simulink model "ssc_car_fuel_cell_1motor"  (R2026a)
settings: Solver=daessc  StopTime=195  FixedStep=1e-3  AbsTol=1e-3
InitFcn:
  | %Vehicle = sm_car_vehcfg_checkConfig(Vehicle);
undefined symbols (not defined in the file): Control, Driver, Init, Maneuver1, Vehicle
libraries: fl_lib x93, nesl_utility x38, GasN_lib x21, sdl_lib x10, simulink_extras x6, SimscapeFluids_lib x6, simulink x5, customMath_lib x5, slpidlib x4, ee_lib x3, autolibshared x2, sl_discontinuities x2
(part 1 of 4)
Description:
  | Vehicle with Fuel Cell Powertrain
  | 
  | Copyright 2020-2025 The MathWorks, Inc.
settings Model: PauseTimes=10  Creator=jrodgers  LastModifiedBy=smiller
settings SolverCC: MaxConsecutiveMinStep=5  SolverJacobianMethodControl=SparsePerturbation  DaesscMode=Fast
settings DataIOCC: SaveFormat=StructureWithTime  SignalLoggingName=logsout_ssc_FuelCell1Motor  ReturnWorkspaceOutputsName=dataOut
settings DebuggingCC: IgnoredZcDiagnostic=none
settings SimscapeCC: SimscapeNominalValues="[{\"value\":\"1\",\"unit\":\"A\"},{\"value\":\"1\",\"unit\":\"bar\"},{\"value\":\"1\",\"unit\":\"cm^2\"},{\"value\":\"1\",\"unit\":\"cm^3/s\"},{\"value\":\"5e6\",\"unit\":\"J/kg\"},{\"value\":\"1\",\"unit\":\"kW\"},{\"value\":\"1\",\"unit\":\"l\"},{\"value\":\"1\",\"unit\":\"N\"},{\"value\":\"1\",\"unit\":\"N*m\"},{\"value\":\"400\",\"unit\":\"V\"},{\"value\":\"355\",\"unit\":\"K\"}]"  SimscapeLogSimulationStatistics=on  SimscapeLogName=simlog_ssc_FuelCell1Motor  SimscapeLogLimitData=off  SimscapeLogDataHistory=5000.0  SimscapeOperatingPoint=ssc_FuelCell1Motor_op10sec

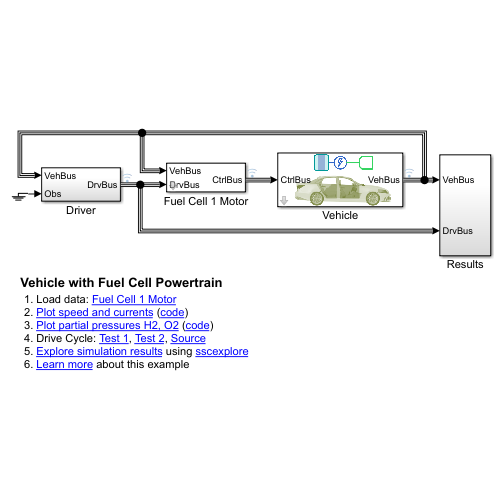
[thumbnail: Simulink's stored preview of the top-level diagram]
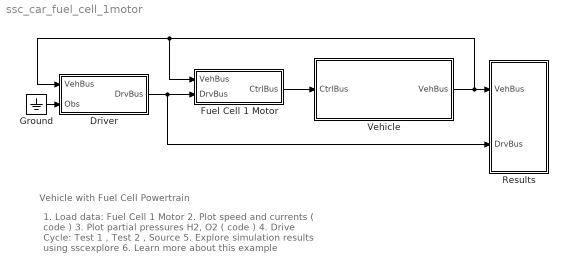
== system ssc_car_fuel_cell_1motor ==
  note: Vehicle with Fuel Cell Powertrain
  note: 1. Load data: Fuel Cell 1 Motor
      | 2. Plot speed and currents ( code )
      | 3. Plot partial pressures H2, O2 ( code )
      | 4. Drive Cycle: Test 1 , Test 2 , Source
      | 5. Explore simulation results using sscexplore
      | 6. Learn more about this example
  Driver : Subsystem  VariantControl=Drive_Cycle
  Fuel Cell 1 Motor : Subsystem  VariantControl=FuelCell1Motor  mask(Control of Fuel Cell Powertrain){Control=Control.FuelCell1Motor}
      mask prompts: Control "Control (structure)"
      mask help: Models control algorithm for fuel cell and regenerative braking of single motor powertrain.
  Ground : Ground
  Results : Subsystem
  Vehicle : Subsystem  mask{Vehicle=Vehicle}
      mask prompts: Vehicle "Vehicle (Structure)"
      mask Display: image('ssc_vehicle_fuel_cell_1motor_vehicle_IMAGE.png');
  wires:
  Vehicle/1(VehBus) -> Fuel Cell 1 Motor/1(VehBus), Driver/1(VehBus), Results/1(VehBus)
  Fuel Cell 1 Motor/1(CtrlBus) -> Vehicle/1(CtrlBus)
  Ground/1 -> Driver/2(Obs)
  Driver/1(DrvBus) -> Fuel Cell 1 Motor/2(DrvBus), Results/2(DrvBus)

== system ssc_car_fuel_cell_1motor/Driver ==
  In Bus Element : Inport  PortName=VehBus  Element=Chassis.Body.CG.vx
  Obs : Inport  Port=2
  Bus Creator2 : BusCreator  Inputs=4
  Constant1 : Constant  Value=0
  Drive Cycle : Subsystem  Variant=on  VariantControlMode=label  VariantControl=Choice  LabelModeActiveChoice=Data
      settings: AttributesFormatString=%<LabelModeActiveChoice>
      mask Display: disp(' ');
  Reference : Subsystem
  Terminator1 : Terminator
  Vehicle Speed Controller : Subsystem  Variant=on  VariantControlMode=label  VariantControl=Choice  LabelModeActiveChoice=Ideal  mask(Driver Model){popup_drivertype=Ideal}
      mask prompts: popup_drivertype "Driver Type"
      mask help: Select from two options. "Ideal" is a simple PI controller. "Configurable" uses the Longitudinal Driver block from Powertrain Blockset which can be configured to include more advanced driver behavior.
      mask init:
      | set_param(gcb,'LabelModeActiveChoice',get_param(gcb,'popup_drivertype'));
      settings: AttributesFormatString=%<LabelModeActiveChoice>
      mask TypeOptions popup_drivertype: Ideal | Configurable
  DrvBus : Outport  VectorParamsAs1DForOutWhenUnconnected=off
  wires:
  Reference/1(Ref) -> Bus Creator2/1  "Reference"
  Constant1/1 -> Bus Creator2/4  "aSteerWheel"
  Bus Creator2/1 -> DrvBus/1
  Obs/1 -> Terminator1/1
  Drive Cycle/1(Reference Speed) -> Reference/1(vTarget), Vehicle Speed Controller/1(Ref Spd)  "vTarget"
  In Bus Element/1 -> Vehicle Speed Controller/2(Veh Spd)
  Vehicle Speed Controller/1(rBrakePedal) -> Bus Creator2/2
  Vehicle Speed Controller/2(rAccelPedal) -> Bus Creator2/3

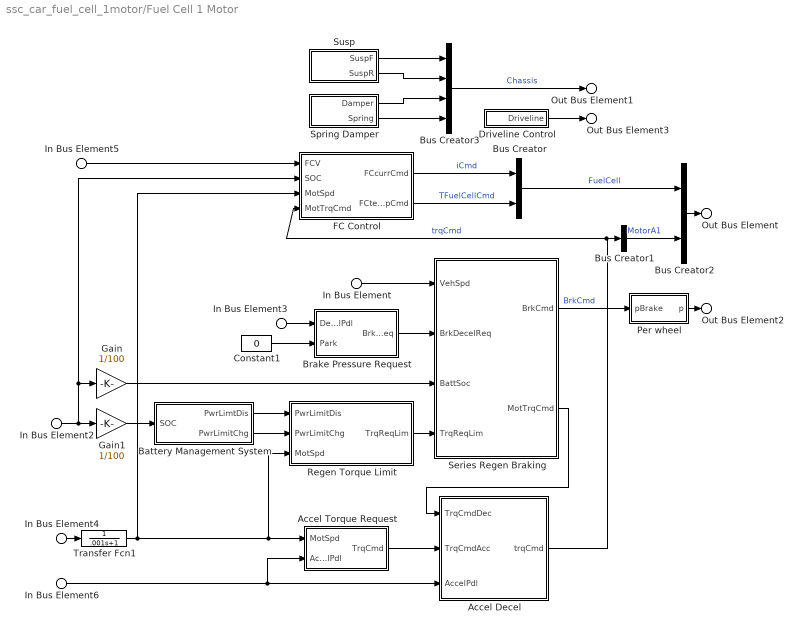
== system ssc_car_fuel_cell_1motor/Fuel Cell 1 Motor ==
  In Bus Element : Inport  PortName=VehBus  Element=Chassis.Body.CG.vx
  In Bus Element2 : Inport  PortName=VehBus  Element=Power.Battery.SOC
  In Bus Element5 : Inport  PortName=VehBus  Element=Power.FuelCell.v
  In Bus Element4 : Inport  PortName=VehBus  Element=Power.MotorA1.w
  In Bus Element3 : Inport  Port=2  PortName=DrvBus  Element=rBrakePedal
  In Bus Element6 : Inport  Port=2  PortName=DrvBus  Element=rAccelPedal
  Accel Decel : Subsystem
  Accel Torque Request : Subsystem
  Battery Management System : Subsystem
  Brake Pressure Request : Subsystem
  Bus Creator : BusCreator  Inputs=2
  Bus Creator1 : BusCreator  Inputs=1
  Bus Creator2 : BusCreator  Inputs=2
  Bus Creator3 : BusCreator  Inputs=4
  Constant1 : Constant  Value=0
  Driveline Control : Subsystem
  FC Control : Subsystem
  Gain : Gain  Gain=1/100
  Gain1 : Gain  Gain=1/100
  Per wheel : Subsystem
  Regen Torque Limit : Subsystem
  Series Regen Braking : Subsystem  InitFcn=%[~]=autosharedicon('autolibutils',gcb,0);  VariantControl=Variant
  Spring Damper : Subsystem
  Susp : Subsystem
  Transfer Fcn1 : TransferFcn  Denominator=[.001 1]
  Out Bus Element : Outport  PortName=CtrlBus  Element=Power
  Out Bus Element2 : Outport  PortName=CtrlBus  Element=Brakes
  Out Bus Element1 : Outport  PortName=CtrlBus  Element=Chassis
  Out Bus Element3 : Outport  PortName=CtrlBus  Element=Driveline
  wires:
  Battery Management System/2(PwrLimitChg) -> Regen Torque Limit/2("PwrLimitChg ")
  Battery Management System/1(PwrLimtDis) -> Regen Torque Limit/1(PwrLimitDis)
  Brake Pressure Request/1(BrkDecelReq) -> Series Regen Braking/2(BrkDecelReq)
  Constant1/1 -> Brake Pressure Request/2(Park)
  In Bus Element/1 -> Series Regen Braking/1(VehSpd)
  Regen Torque Limit/1("TrqReqLim ") -> Series Regen Braking/4(TrqReqLim)
  Accel Torque Request/1(TrqCmd) -> Accel Decel/2(TrqCmdAcc)
  Per wheel/1(p) -> Out Bus Element2/1
  Series Regen Braking/1(" BrkCmd") -> Per wheel/1(pBrake)  "BrkCmd"
  Series Regen Braking/2(" MotTrqCmd") -> Accel Decel/1(TrqCmdDec)
  Driveline Control/1(Driveline) -> Out Bus Element3/1
  Susp/2(SuspR) -> Bus Creator3/2
  Spring Damper/2(Spring) -> Bus Creator3/4
  Bus Creator3/1 -> Out Bus Element1/1  "Chassis"
  Susp/1(SuspF) -> Bus Creator3/1
  Spring Damper/1(Damper) -> Bus Creator3/3
  Transfer Fcn1/1 -> FC Control/3(MotSpd), Accel Torque Request/1(MotSpd), Regen Torque Limit/3(MotSpd)
  Bus Creator2/1 -> Out Bus Element/1
  Bus Creator1/1 -> Bus Creator2/2  "MotorA1"
  Bus Creator/1 -> Bus Creator2/1  "FuelCell"
  FC Control/1(FCcurrCmd) -> Bus Creator/1  "iCmd"
  In Bus Element5/1 -> FC Control/1(FCV)
  FC Control/2(FCtempCmd) -> Bus Creator/2  "TFuelCellCmd"
  In Bus Element2/1 -> Gain1/1, Gain/1, FC Control/2(SOC)
  In Bus Element3/1 -> Brake Pressure Request/1(DecelPdl)
  Gain/1 -> Series Regen Braking/3(BattSoc)
  In Bus Element4/1 -> Transfer Fcn1/1
  Gain1/1 -> Battery Management System/1(SOC)
  In Bus Element6/1 -> Accel Decel/3(AccelPdl), Accel Torque Request/2(AccelPdl)
  Accel Decel/1(trqCmd) -> Bus Creator1/1, FC Control/4(MotTrqCmd)  "trqCmd"

== system ssc_car_fuel_cell_1motor/Results ==
  In Bus Element3 : Inport  PortName=VehBus
  In Bus Element2 : Inport  PortName=VehBus  Element=Power.FuelCell.i
  In Bus Element1 : Inport  PortName=VehBus  Element=Power.Battery.Power
  DrvBus : Inport  Port=2
  Bus Selector : BusSelector  OutputSignals=Reference.vTarget
  Bus Selector1 : BusSelector  OutputSignals=Chassis.Body.CG.vx
  Fuel Economy : Subsystem
  Scope : Scope  NumInputPorts=2
      settings: ActiveDisplayYMinimum=-3.42768  ActiveDisplayYMaximum=28.54488
  Scope1 : Scope  NumInputPorts=2
      settings: ActiveDisplayYMinimum=-12.71615  ActiveDisplayYMaximum=114.44535  DataLoggingVariableName=ScopeData2
  wires:
  DrvBus/1 -> Bus Selector/1
  Bus Selector/1 -> Scope/1  "<vTarget>"
  In Bus Element3/1 -> Bus Selector1/1
  Bus Selector1/1 -> Fuel Economy/1(In1), Scope/2  "<vx>"
  In Bus Element2/1 -> Fuel Economy/2(In2)
  In Bus Element1/1 -> Fuel Economy/3(In3)
  Fuel Economy/1(MPGe) -> Scope1/1  "MPGe"
  Fuel Economy/2(l/100km) -> Scope1/2  "Liters/100km"

== system ssc_car_fuel_cell_1motor/Vehicle ==
  In Bus Element : Inport  PortName=CtrlBus  Element=Power
  In Bus Element2 : Inport  PortName=CtrlBus  Element=Brakes
  Chassis : Subsystem  VariantControl=Full
      mask Display: image('ssc_vehicle_fuel_cell_1motor_chassis_IMAGE.png');
  Powertrain : Subsystem  mask{Powertrain=Vehicle.Powertrain}
      mask prompts: Powertrain "Powertrain (structure)"
      mask Display: image('ssc_vehicle_fuel_cell_1motor_powertrain_IMAGE.png');
  Solver Configuration : nesl_utility/Solver Configuration  PhysicalDomain=network_engine_domain  SubClassName=solver  LeftPortType=input  RightPortType=generic  Tones=[]  Harmonics=[]  SimulateNoise=off  Profile=off  UseLocalSampling=off  EnableSwitchedLinearOptims=on  FrequencyDomain=off  UseCCode=off  RelTol=0.001  AbsTol=1e-06  MinStep=1e-09  ToWorkspace=off  RevertToSquareIcSolve=off  NumHomotopyIterations=100  PhasorMode=off  PhasorModeNumHarmonics=1  ConsistencySolver=NEWTON_FTOL  CanonicalOrdering=UNORDERED  OptimizeIntermediates=UNOPTIMIZED  IndexReductionMethod=DerivativeReplacement  DoDC=off  ResidualTolerance=1e-09  ConsistencyTolSource=GLOBAL  ConsistencyAbsTol=0.001  ConsistencyRelTol=0.001  ConsistencyTolFactor=0.001  UseLocalSolver=off  LocalSolverChoice=NE_BACKWARD_EULER_ADVANCER  ResolveIndetEquations=on  FunctionEvalNumThread=1  LocalSolverSampleTime=0.001  DoFixedCost=off  MaxNonlinIter=3  MaxModeIter=2  ComputeImpulses=off  ImpulseIterations=2  LinearAlgebra=auto  LinearAlgebraNumThread=0  EquationFormulation=NE_TIME_EF  DelaysMemoryBudget=1024  AutomaticFiltering=on  FilteringTimeConstant=0.001  PartitionStorageMethod=AS_NEEDED  PartitionMemoryBudget=1024  PartitionMethod=FAST  MultibodyUseLocalSolver=off  MultibodyLocalSolverChoice=ODE1  MultibodyLocalSolverSampleTime=0.001
  Out Bus Element : Outport  PortName=VehBus  Element=Power
  Out Bus Element1 : Outport  PortName=VehBus  Element=Chassis
  wires:
  Powertrain/1(OutP) -> Out Bus Element/1
  In Bus Element2/1 -> Chassis/1(Brakes)
  In Bus Element/1 -> Powertrain/2(CtrlP)
  Chassis/1(VehBus) -> Powertrain/1(VehB), Out Bus Element1/1
  connections:
  Chassis/RConn1 -- Powertrain/RConn1
  Powertrain/LConn1 -- Chassis/LConn1 -- Solver Configuration/RConn1

== system ssc_car_fuel_cell_1motor/Driver/Drive Cycle ==
  Drive Cycle Data : Subsystem  VariantControl=Data  mask{popup_cycle=Cycle 1, Drive_Cycle_Time=Maneuver1.DriveCycle.cycle_t.Value, Drive_Cycle_Speed=Maneuver1.DriveCycle.cycle_spd.Value}
      mask prompts: popup_cycle "Drive Cycle"; Drive_Cycle_Time "Drive Cycle Time (s)"; Drive_Cycle_Speed "Drive Cycle Speed (km/h)"
      mask init:
      | if(verLessThan('matlab','9.7'))
      |     set_param([gcb '/1-D Lookup Table'],'InterpMethod','Cubic spline')
      | else
      |     set_param([gcb '/1-D Lookup Table'],'InterpMethod','Akima spline')
      | end
      mask TypeOptions popup_cycle: Cycle 1 | Cycle 2 | Custom
      mask Callback popup_cycle:
      | maskObj = Simulink.Mask.get(gcb);
      | dct_h = maskObj.getParameter('Drive_Cycle_Time');
      | dcs_h = maskObj.getParameter('Drive_Cycle_Speed');
      | 
      | if strcmp(get_param(gcb,'popup_cycle'),'Cycle 1')
      |     dct_h.Value = 'Maneuver1.DriveCycle.cycle_t.Value';
      |     dcs_h.Value = 'Maneuver1.DriveCycle.cycle_spd.Value';
      |     dct_h.Enabled = 'off';
      |     dcs_h.Enabled = 'off';
      | elseif strcmp(get_param(gcb,'popup_cycle'),'Cycle 2')
      |     dct_h.Value = 'Maneuver2.DriveCycle.cycle_t.Value';
      |     dcs_h.Value = 'Maneuver2.DriveCycle.cycle_spd.Value';
      |     dct_h.Enabled = 'off';
      |     dcs_h.Enabled = 'off';
      | elseif strcmp(get_param(gcb,'popup_cycle'),'Custom')
      |     dct_h.Enabled = 'on';
      |     dcs_h.Enabled = 'on';
      | end
      | 
      | clear maskObj dct_h dcs_h
  Drive Cycle Source : autolibshared/Drive Cycle Source  VariantControl=Source  cycleVar=FTP75  fileVar=cycleFTP75.mat  tfinal="2474  seconds"  cycleRepeat=off  outAccPort=off  outGearPort=off  gearList=No gear data  t_wot1=5  xdot_woto=0  xdot_wot1=30  t_wot2=20  xdot_wot2=0  t_wotend=30  srcUnit=m/s  outUnit=m/s  srcAccUnit=m/s/s  outAccUnit=m/s^2  dt=0  aMode=1  faultOption=off  velBnd=2  velBndUnit=mph  inUnit=m/s  timeBnd=1  failOption=off  stopSim=off  maxFaultCnt=10  maxFaultTime=2  maxTotFaultTime=15  traceOption=off  dtTrace=1  traceWindow=10  lastDCname=FTP75  lastOutUnit=mph  lastDT=0  lastTB=1  lastSB=2  forceCalcBound=off
  Reference Speed : Outport

== system ssc_car_fuel_cell_1motor/Driver/Reference ==
  vTarget : Inport
  Bus Creator : BusCreator  Inputs=5
  Constant2 : Constant  Value=0
  Constant4 : Constant  Value=0
  Gain : Gain
  Integrator : Integrator
  Ref : Outport  VectorParamsAs1DForOutWhenUnconnected=off
  wires:
  Bus Creator/1 -> Ref/1
  Constant2/1 -> Bus Creator/3  "y"
  Gain/1 -> Bus Creator/1  "dist"
  Integrator/1 -> Gain/1, Bus Creator/2  "x"
  Constant4/1 -> Bus Creator/4  "aYaw"
  vTarget/1 -> Integrator/1, Bus Creator/5

== system ssc_car_fuel_cell_1motor/Driver/Vehicle Speed Controller ==
  Ref Spd : Inport
  Veh Spd : Inport  Port=2
  Configurable : Subsystem  VariantControl=Configurable
  Ideal : Subsystem  VariantControl=Ideal  mask(PI Controller){Driver=Driver}
      mask prompts: Driver "Driver (structure)"
      mask help: Simple PI controller to follow reference signal.
  rBrakePedal : Outport
  rAccelPedal : Outport  Port=2

== system ssc_car_fuel_cell_1motor/Fuel Cell 1 Motor/Accel Decel ==
  TrqCmdDec : Inport
  TrqCmdAcc : Inport  Port=2
  AccelPdl : Inport  Port=3
  Accel Decel Switch : Switch  Criteria=u2 > Threshold  SaturateOnIntegerOverflow=off  InputSameDT=off
  Compare To Constant : simulink/Logic and Bit Operations/Compare To Constant  relop=>  const=1e-3  OutDataTypeStr=boolean  ZeroCross=off
  trqCmd : Outport  VectorParamsAs1DForOutWhenUnconnected=off
  wires:
  Compare To Constant/1 -> Accel Decel Switch/2
  AccelPdl/1 -> Compare To Constant/1
  TrqCmdAcc/1 -> Accel Decel Switch/1
  Accel Decel Switch/1 -> trqCmd/1
  TrqCmdDec/1 -> Accel Decel Switch/3

== system ssc_car_fuel_cell_1motor/Fuel Cell 1 Motor/Accel Torque Request ==
  note: Convert Accelerator Pedal Position to Torque Command
      | using Motor Torque Speed Curve
  MotSpd : Inport
  AccelPdl : Inport  Port=2
  MaxMotTrqVsSpd : Lookup_n-D  NumberOfTableDimensions=1  BreakpointsForDimension1=Control.MotorA1.TorqueSpd.w.Value %Mot.w_eff_bp_EV_rear  Table=Control.MotorA1.TorqueSpd.trq.Value % Mot.T_t_EV_rear  ExtrapMethod=Clip  UseLastTableValue=on  InternalRulePriority=Speed  OutDataTypeStr=Inherit: Inherit from 'Table data'  RndMeth=Simplest
  Product1 : Product
  rads_to_rpm : Gain  Gain=30/pi
  TrqCmd : Outport  VectorParamsAs1DForOutWhenUnconnected=off
  wires:
  Product1/1 -> TrqCmd/1
  MaxMotTrqVsSpd/1 -> Product1/2
  AccelPdl/1 -> Product1/1
  MotSpd/1 -> rads_to_rpm/1
  rads_to_rpm/1 -> MaxMotTrqVsSpd/1

== system ssc_car_fuel_cell_1motor/Fuel Cell 1 Motor/Battery Management System ==
  note: Behaviorial BMS System. Limits battery charge / discharge power based on SOC.
      |
      | Charge/Discharge Limits and curves can be adjusted if using a larger battery pack
      | or motor power is changed.
  SOC : Inport
  ChrgLmt : Lookup_n-D  NumberOfTableDimensions=1  BreakpointsForDimension1=Control.Battery.SOC_bpt  Table=Control.Battery.ChrgLmt_bpt  ExtrapMethod=Clip  UseLastTableValue=on  InternalRulePriority=Speed  RndMeth=Simplest
  DischrgLmt : Lookup_n-D  NumberOfTableDimensions=1  BreakpointsForDimension1=Control.Battery.SOC_bpt  Table=Control.Battery.DischrgLmt_bpt  ExtrapMethod=Clip  UseLastTableValue=on  InternalRulePriority=Speed  RndMeth=Simplest
  MaxChrg : Constant  Value=Control.Battery.BattChrgMax
  MaxDischrg : Constant  Value=Control.Battery.BattDischrgMax
  Product : Product
  Product1 : Product
  PwrLimtDis : Outport  VectorParamsAs1DForOutWhenUnconnected=off
  PwrLimitChg : Outport  Port=2  VectorParamsAs1DForOutWhenUnconnected=off
  wires:
  SOC/1 -> DischrgLmt/1, ChrgLmt/1
  MaxChrg/1 -> Product1/2
  MaxDischrg/1 -> Product/2
  Product/1 -> PwrLimtDis/1
  Product1/1 -> PwrLimitChg/1
  ChrgLmt/1 -> Product1/1
  DischrgLmt/1 -> Product/1

== system ssc_car_fuel_cell_1motor/Fuel Cell 1 Motor/Brake Pressure Request ==
  note: Converts Brake Pedal Position to Deceleration Request
  DecelPdl : Inport
  Park : Inport  Port=2
  Constant1 : Constant
  Switch : Switch  Criteria=u2 > Threshold  ZeroCross=off  SaturateOnIntegerOverflow=off  InputSameDT=off
  BrkDecelReq : Outport  VectorParamsAs1DForOutWhenUnconnected=off
  wires:
  DecelPdl/1 -> Switch/3
  Constant1/1 -> Switch/1
  Switch/1 -> BrkDecelReq/1
  Park/1 -> Switch/2

== system ssc_car_fuel_cell_1motor/Fuel Cell 1 Motor/Driveline Control ==
  Bus Creator : BusCreator  Inputs=1
  Constant : Constant  Value=0
  Driveline : Outport  VectorParamsAs1DForOutWhenUnconnected=off
  wires:
  Constant/1 -> Bus Creator/1  "placeholder"
  Bus Creator/1 -> Driveline/1  "Driveline"

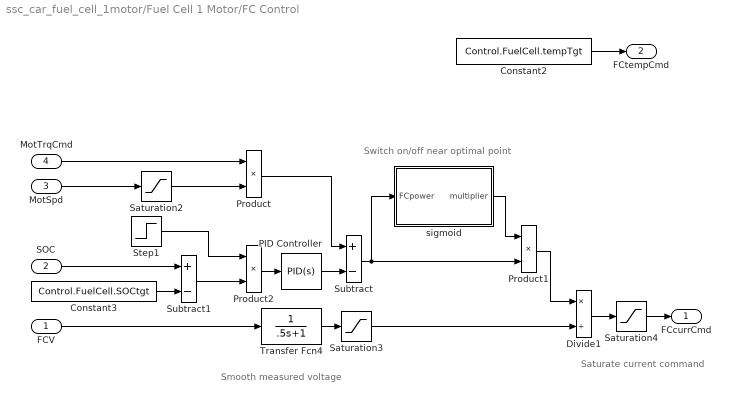
== system ssc_car_fuel_cell_1motor/Fuel Cell 1 Motor/FC Control ==
  note: Saturate current command
  note: Smooth measured voltage
  note: Switch on/off near optimal point
  FCV : Inport
  SOC : Inport  Port=2
  MotSpd : Inport  Port=3
  MotTrqCmd : Inport  Port=4
  Constant2 : Constant  Value=Control.FuelCell.tempTgt
  Constant3 : Constant  Value=Control.FuelCell.SOCtgt
  Divide1 : Product  Inputs=*/
  PID Controller : slpidlib/PID Controller  Controller=PID  Form=Parallel  TimeDomain=Continuous-time  UseExternalTs=off  SampleTime=-1  IntegratorMethod=Forward Euler  FilterMethod=Forward Euler  ControllerParametersSource=internal  P=10000/100  I=0  UseKiTs=off  D=0  UseExternalDerivativeSource=off  N=100  UseFilter=on  TunerSelectOption=Transfer Function Based (PID Tuner App)  ZeroCross=off  InitialConditionSource=internal  InitialConditionForIntegrator=0  InitialConditionForFilter=0  DifferentiatorICPrevScaledInput=0  ExternalReset=none  TrackingMode=off  Kt=1  LimitOutput=off  SatLimitsSource=internal  UpperSaturationLimit=inf  LowerSaturationLimit=-inf  LinearizeAsGain=on  AntiWindupMode=none  Kb=1  LimitIntegrator=off  UpperIntegratorSaturationLimit=inf  LowerIntegratorSaturationLimit=-inf  POutMin=[]  POutMax=[]  IOutMin=[]  IOutMax=[]  DOutMin=[]  DOutMax=[]  NOutMin=[]  NOutMax=[]  SumOutMin=[]  SumOutMax=[]  SaturationOutMin=[]  SaturationOutMax=[]  PParamMin=[]  PParamMax=[]  IParamMin=[]  IParamMax=[]  DParamMin=[]  DParamMax=[]  NParamMin=[]  NParamMax=[]  KbParamMin=[]  KbParamMax=[]  KtParamMin=[]  KtParamMax=[]  KbOutMin=[]  KbOutMax=[]  KtOutMin=[]  KtOutMax=[]  IntegratorOutMin=[]  IntegratorOutMax=[]  FilterOutMin=[]  FilterOutMax=[]  SumI1OutMin=[]  SumI1OutMax=[]  SumI2OutMin=[]  SumI2OutMax=[]  SumI3OutMin=[]  SumI3OutMax=[]  SumI4OutMin=[]  SumI4OutMax=[]  SumDOutMin=[]  SumDOutMax=[]  DifferentiatorOutMin=[]  DifferentiatorOutMax=[]  FilterDiffOutCoefMin=[]  FilterDiffOutCoefMax=[]  ReciprocalOutMin=[]  ReciprocalOutMax=[]  SumDenOutMin=[]  SumDenOutMax=[]  SumNumOutMin=[]  SumNumOutMax=[]  DivideOutMin=[]  DivideOutMax=[]  UdiffTsProdOutMin=[]  UdiffTsProdOutMax=[]  NTsProdOutMin=[]  NTsProdOutMax=[]  UintegralTsProdOutMin=[]  UintegralTsProdOutMax=[]  UngainTsProdOutMin=[]  UngainTsProdOutMax=[]  ClampingZeroOutDataTypeStr=Inherit: Inherit via back propagation  ClampingZeroOutMin=[]  ClampingZeroOutMax=[]  FilterDenConstantOutDataTypeStr=Inherit: Inherit via back propagation  FilterDenConstantOutMin=[]  FilterDenConstantOutMax=[]  PCopyOutDataTypeStr=Inherit: Inherit via back propagation  PCopyOutMin=[]  PCopyOutMax=[]  NCopyOutDataTypeStr=Inherit: Inherit via back propagation  NCopyOutMin=[]  NCopyOutMax=[]  IntegratorContinuousStateAttributes=''  IntegratorStateMustResolveToSignalObject=off  IntegratorRTWStateStorageClass=Auto  FilterContinuousStateAttributes=''  FilterStateMustResolveToSignalObject=off  FilterRTWStateStorageClass=Auto  ParallelPVariant=InternalParameters  IdealPVariant=Disabled  IVariant=InternalParameters  DVariant=InternalParameters  IntegratorVariant=Continuous  SatVariant=Disabled  AWVariant=Passthrough  PCopyVariant=Disabled  TRVariant=Disabled  FdbkBlocksVariant=Forward  IdealPFdbkVariant=Disabled  SatFdbkVariant=Disabled  DerivativeFilterVariant=ContFilter  NVariant=InternalParameters  NCopyVariant=Disabled  FilterICVariant=InternalICsFilter  IntegratorICVariant=InternalICs  ExternalResetVariant=Disabled  TRSumVariant=Passthrough  SumFdbkVariant=Disabled  SumVariant=Sum_PID  TsampFilterVariant=InternalTs  TsampNgainVariant=Passthrough  TsampIntegralVariant=Disabled_SignalSpec  ExternalSaturationOutDataTypeStr=Inherit: Same as second input  DerivativeSourceVariant=ErrorSignal  PreIntVariant=InternalPreInt
  Product : Product
  Product1 : Product
  Product2 : Product
  Saturation2 : Saturate  UpperLimit=inf  LowerLimit=1  ZeroCross=off
  Saturation3 : Saturate  UpperLimit=inf  LowerLimit=200  ZeroCross=off
  Saturation4 : Saturate  UpperLimit=350  LowerLimit=0  ZeroCross=off
  Step1 : Step  SampleTime=0
  Subtract : Sum  Inputs=+-
  Subtract1 : Sum  Inputs=+-
  Transfer Fcn4 : TransferFcn  Denominator=[.5 1]
  sigmoid : Subsystem
  FCcurrCmd : Outport
  FCtempCmd : Outport  Port=2
  wires:
  Subtract/1 -> sigmoid/1(FCpower), Product1/2
  sigmoid/1(multiplier) -> Product1/1
  Product1/1 -> Divide1/1
  Product/1 -> Subtract/1
  Product2/1 -> PID Controller/1
  Constant2/1 -> FCtempCmd/1
  MotSpd/1 -> Saturation2/1
  Subtract1/1 -> Product2/2
  MotTrqCmd/1 -> Product/1
  Saturation2/1 -> Product/2
  Divide1/1 -> Saturation4/1
  FCV/1 -> Transfer Fcn4/1
  Saturation4/1 -> FCcurrCmd/1
  Constant3/1 -> Subtract1/2
  Step1/1 -> Product2/1
  SOC/1 -> Subtract1/1
  Saturation3/1 -> Divide1/2
  Transfer Fcn4/1 -> Saturation3/1
  PID Controller/1 -> Subtract/2

== system ssc_car_fuel_cell_1motor/Fuel Cell 1 Motor/Per wheel ==
  pBrake : Inport
  Bus Creator4 : BusCreator  Inputs=4
  Gain1 : Gain  Gain=0.6
  Gain2 : Gain  Gain=0.6
  Gain3 : Gain  Gain=0.4
  Gain4 : Gain  Gain=0.4
  Gain5 : Gain  Gain=0.5
  Transfer Fcn : TransferFcn  Denominator=[0.01 1]
  p : Outport  VectorParamsAs1DForOutWhenUnconnected=off
  wires:
  Transfer Fcn/1 -> Gain5/1
  Gain5/1 -> Gain4/1, Gain3/1, Gain1/1, Gain2/1  "pBrakeL1"
  Gain2/1 -> Bus Creator4/1  "pBrakeL1"
  pBrake/1 -> Transfer Fcn/1
  Bus Creator4/1 -> p/1
  Gain1/1 -> Bus Creator4/2  "pBrakeR1"
  Gain3/1 -> Bus Creator4/3  "pBrakeL2"
  Gain4/1 -> Bus Creator4/4  "pBrakeR2"

== system ssc_car_fuel_cell_1motor/Fuel Cell 1 Motor/Regen Torque Limit ==
  note: Power Management algorithm:
      | - Estimate Elec power based on mech power using efficiency map
      | - Check if Elec power is within battery power limits
      | - If power within limit , use motor torque command
      | - If power limit exceeded, use limited motor torque
      | - For low Mot Spd, MotPwrReq will be a small number.  Pass through torque command until Mot Spd > 2.
  PwrLimitDis : Inport
  "PwrLimitChg " : Inport  Port=2
  MotSpd : Inport  Port=3
  Abs : Abs  ZeroCross=off  SaturateOnIntegerOverflow=off
  Check Within Limits : Subsystem
  Compare To Constant1 : simulink/Logic and Bit Operations/Compare To Constant  relop=<  const=2  OutDataTypeStr=boolean  ZeroCross=off
  ElecToMechPwr : Product  Inputs=*/
  Gain : Gain  Gain=-1
  MaxMotTrqVsSpd : Lookup_n-D  NumberOfTableDimensions=1  BreakpointsForDimension1=Control.MotorA1.TorqueSpd.w.Value  Table=Control.MotorA1.TorqueSpd.trq.Value  ExtrapMethod=Clip  UseLastTableValue=on  InternalRulePriority=Speed  OutDataTypeStr=Inherit: Inherit from 'Table data'  RndMeth=Simplest
  Mech to Elec Power Estimate : Subsystem
  MechPwrToTrq : Product  Inputs=*/
  Saturation : Saturate  UpperLimit=inf  LowerLimit=2
  Switch : Switch  Criteria=u2 > Threshold  ZeroCross=off  SaturateOnIntegerOverflow=off  InputSameDT=off
  Switch1 : Switch  Criteria=u2 > Threshold  ZeroCross=off  SaturateOnIntegerOverflow=off  InputSameDT=off
  Torque Limit : Subsystem
  rads_to_rpm : Gain  Gain=30/pi
  "TrqReqLim " : Outport  VectorParamsAs1DForOutWhenUnconnected=off
  wires:
  MotSpd/1 -> rads_to_rpm/1, Mech to Elec Power Estimate/2(MotSpd), Saturation/1, Abs/1, Torque Limit/2(MotSpd)
  MaxMotTrqVsSpd/1 -> Gain/1  "MotTrqMax"
  rads_to_rpm/1 -> MaxMotTrqVsSpd/1
  ElecToMechPwr/1 -> MechPwrToTrq/1
  MechPwrToTrq/1 -> Switch/3
  Saturation/1 -> MechPwrToTrq/2
  Compare To Constant1/1 -> Switch1/2
  Abs/1 -> Compare To Constant1/1
  Switch/1 -> Switch1/3
  Mech to Elec Power Estimate/1(MotPwrElecReq) -> Check Within Limits/2(u)
  Check Within Limits/2(y) -> ElecToMechPwr/1
  Check Within Limits/1(InLimit) -> Switch/2
  Gain/1 -> Switch/1, Switch1/1, Mech to Elec Power Estimate/1(MotTrqCmd)
  "PwrLimitChg "/1 -> Check Within Limits/3(lo)
  PwrLimitDis/1 -> Check Within Limits/1(up)
  Mech to Elec Power Estimate/2(Eff2k) -> ElecToMechPwr/2
  Torque Limit/1(MotReqCmd) -> "TrqReqLim "/1
  Switch1/1 -> Torque Limit/1(MotTrq)

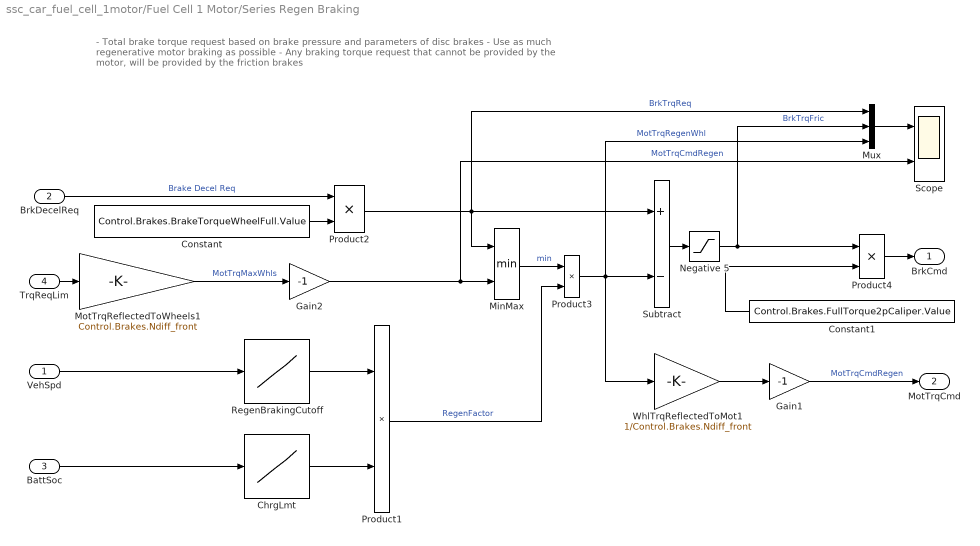
== system ssc_car_fuel_cell_1motor/Fuel Cell 1 Motor/Series Regen Braking ==
  note: - Total brake torque request based on brake pressure and parameters of disc brakes
      | - Use as much regenerative motor braking as possible
      | - Any braking torque request that cannot be provided by the motor, will be provided by the friction brakes
  VehSpd : Inport
  BrkDecelReq : Inport  Port=2
  BattSoc : Inport  Port=3
  TrqReqLim : Inport  Port=4
  ChrgLmt : Lookup_n-D  NumberOfTableDimensions=1  BreakpointsForDimension1=Control.Battery.SOC_bpt  Table=Control.Battery.ChrgLmt_bpt  ExtrapMethod=Clip  UseLastTableValue=on  InternalRulePriority=Speed  RndMeth=Simplest
  Constant : Constant  Value=Control.Brakes.BrakeTorqueWheelFull.Value
  Constant1 : Constant  Value=Control.Brakes.FullTorque2pCaliper.Value
  Gain1 : Gain  Gain=-1
  Gain2 : Gain  Gain=-1
  MinMax : MinMax  Inputs=2
  MotTrqReflectedToWheels1 : Gain  Gain=Control.Brakes.Ndiff_front
  Mux : Mux  Inputs=3
  Negative 5 : Saturate  UpperLimit=inf  LowerLimit=0  ZeroCross=off
  Product1 : Product
  Product2 : Product
  Product3 : Product
  Product4 : Product  Inputs=**
  RegenBrakingCutoff : Lookup_n-D  NumberOfTableDimensions=1  BreakpointsForDimension1=Control.Power.RegenBrkSpd_bpt  Table=Control.Power.RegenBrkCutOff  ExtrapMethod=Clip  UseLastTableValue=on  InternalRulePriority=Speed  RndMeth=Simplest
  Scope : Scope  NumInputPorts=2
      settings: ActiveDisplayYMinimum=-294.72625  ActiveDisplayYMaximum=2652.53625
  Subtract : Sum  Inputs=+-
  WhlTrqReflectedToMot1 : Gain  Gain=1/Control.Brakes.Ndiff_front
  " BrkCmd" : Outport  VectorParamsAs1DForOutWhenUnconnected=off
  " MotTrqCmd" : Outport  Port=2  VectorParamsAs1DForOutWhenUnconnected=off
  wires:
  MotTrqReflectedToWheels1/1 -> Gain2/1  "MotTrqMaxWhls"
  Gain2/1 -> Scope/2, MinMax/2  "MotTrqCmdRegen"
  Gain1/1 -> " MotTrqCmd"/1  "MotTrqCmdRegen"
  WhlTrqReflectedToMot1/1 -> Gain1/1
  TrqReqLim/1 -> MotTrqReflectedToWheels1/1
  Mux/1 -> Scope/1
  Product3/1 -> Mux/3, Subtract/2, WhlTrqReflectedToMot1/1  "MotTrqRegenWhl"
  Constant1/1 -> Product4/2
  Constant/1 -> Product2/2
  BrkDecelReq/1 -> Product2/1  "Brake Decel Req"
  Product2/1 -> Mux/1, Subtract/1, MinMax/1  "BrkTrqReq"
  MinMax/1 -> Product3/1  "min"
  ChrgLmt/1 -> Product1/2
  VehSpd/1 -> RegenBrakingCutoff/1
  RegenBrakingCutoff/1 -> Product1/1
  Product1/1 -> Product3/2  "RegenFactor"
  Subtract/1 -> Negative 5/1
  BattSoc/1 -> ChrgLmt/1
  Negative 5/1 -> Mux/2, Product4/1  "BrkTrqFric"
  Product4/1 -> " BrkCmd"/1

== system ssc_car_fuel_cell_1motor/Fuel Cell 1 Motor/Spring Damper ==
  Bus Creator : BusCreator  Inputs=4
  Bus Creator1 : BusCreator  Inputs=4
  Constant : Constant  Value=[0 0 0 0]
  Constant1 : Constant  Value=[0 0 0 0]
  Demux : Demux
  Demux1 : Demux
  Damper : Outport  VectorParamsAs1DForOutWhenUnconnected=off
  Spring : Outport  Port=2  VectorParamsAs1DForOutWhenUnconnected=off
  wires:
  Bus Creator/1 -> Spring/1  "Spring"
  Bus Creator1/1 -> Damper/1  "Damper"
  Constant1/1 -> Demux1/1
  Demux1/3 -> Bus Creator1/3  "RL"
  Demux1/4 -> Bus Creator1/4  "RR"
  Demux1/1 -> Bus Creator1/1  "FL"
  Demux1/2 -> Bus Creator1/2  "FR"
  Demux/2 -> Bus Creator/2  "FR"
  Demux/1 -> Bus Creator/1  "FL"
  Demux/4 -> Bus Creator/4  "RR"
  Demux/3 -> Bus Creator/3  "RL"
  Constant/1 -> Demux/1

== system ssc_car_fuel_cell_1motor/Fuel Cell 1 Motor/Susp ==
  Bus Creator1 : BusCreator  Inputs=1
  Bus Creator2 : BusCreator  Inputs=1
  Bus Creator3 : BusCreator  Inputs=1
  Constant1 : Constant  Value=0
  Steer : Subsystem
  SuspF : Outport  VectorParamsAs1DForOutWhenUnconnected=off
  SuspR : Outport  Port=2  VectorParamsAs1DForOutWhenUnconnected=off
  wires:
  Steer/1(Steer) -> Bus Creator1/1
  Constant1/1 -> Bus Creator2/1  "iMotor"
  Bus Creator2/1 -> Bus Creator3/1  "Steer"
  Bus Creator3/1 -> SuspR/1  "SuspR"
  Bus Creator1/1 -> SuspF/1  "SuspF"

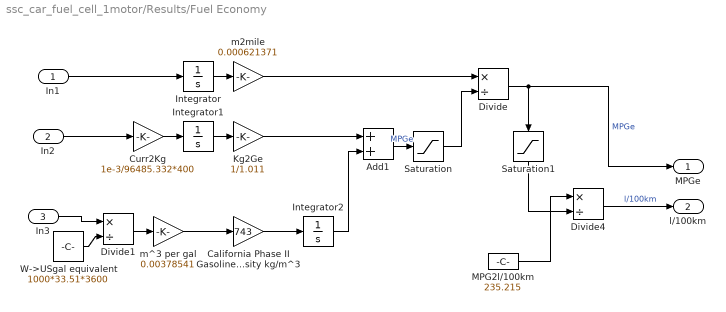
== system ssc_car_fuel_cell_1motor/Results/Fuel Economy ==
  In1 : Inport
  In2 : Inport  Port=2
  In3 : Inport  Port=3
  Add1 : Sum
  California Phase II Gasoline density kg/m^3 : Gain  Gain=743
  Curr2Kg : Gain  Gain=1e-3/96485.332*400
  Divide : Product  Inputs=*/
  Divide1 : Product  Inputs=*/
  Divide4 : Product  Inputs=*/
  Integrator : Integrator
  Integrator1 : Integrator
  Integrator2 : Integrator
  Kg2Ge : Gain  Gain=1/1.011
  MPG2l/100km : Constant  Value=235.215
  Saturation : Saturate  UpperLimit=inf  LowerLimit=0.0001
  Saturation1 : Saturate  UpperLimit=inf  LowerLimit=10
  W->USgal equivalent : Constant  Value=1000*33.51*3600
  m2mile : Gain  Gain=0.000621371
  m^3 per gal : Gain  Gain=0.00378541
  MPGe : Outport  VectorParamsAs1DForOutWhenUnconnected=off
  l/100km : Outport  Port=2  VectorParamsAs1DForOutWhenUnconnected=off
  wires:
  MPG2l/100km/1 -> Divide4/1
  m^3 per gal/1 -> California Phase II Gasoline density kg/m^3/1
  Divide4/1 -> l/100km/1  "l/100km"
  Integrator/1 -> m2mile/1
  Divide/1 -> MPGe/1, Saturation1/1  "MPGe"
  Saturation/1 -> Divide/2
  In2/1 -> Curr2Kg/1
  California Phase II Gasoline density kg/m^3/1 -> Integrator2/1
  Add1/1 -> Saturation/1  "MPGe"
  In1/1 -> Integrator/1
  Integrator2/1 -> Add1/2
  W->USgal equivalent/1 -> Divide1/2
  m2mile/1 -> Divide/1
  Saturation1/1 -> Divide4/2
  Curr2Kg/1 -> Integrator1/1
  Kg2Ge/1 -> Add1/1
  Divide1/1 -> m^3 per gal/1
  Integrator1/1 -> Kg2Ge/1
  In3/1 -> Divide1/1

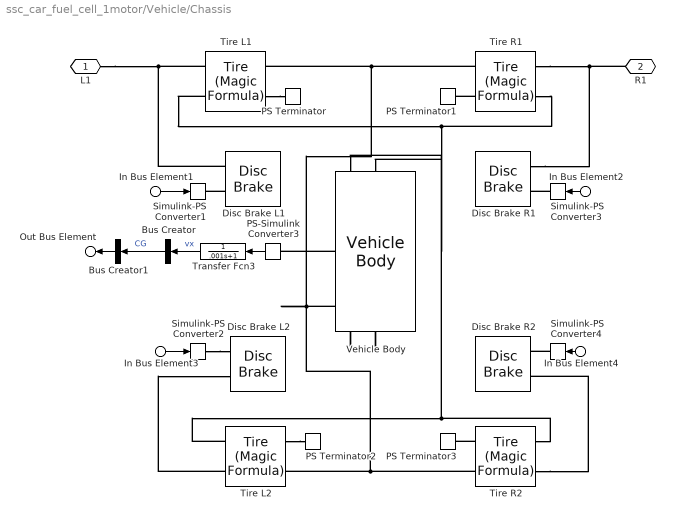
== system ssc_car_fuel_cell_1motor/Vehicle/Chassis ==
  In Bus Element1 : Inport  PortName=Brakes  Element=pBrakeL1
  In Bus Element2 : Inport  PortName=Brakes  Element=pBrakeR1
  In Bus Element3 : Inport  PortName=Brakes  Element=pBrakeL2
  In Bus Element4 : Inport  PortName=Brakes  Element=pBrakeR2
  Bus Creator : BusCreator  Inputs=1
  Bus Creator1 : BusCreator  Inputs=1
  Disc Brake L1 : sdl_lib/Brakes & Detents/Rotational/Disc Brake  r_mean=Vehicle.Brakes.Axle1.DiscAndPad.lMeanRadius.Value m  bore=Vehicle.Brakes.Axle1.Caliper.lCylinderDiameter.Value m  n_pads=Vehicle.Brakes.Axle1.DiscAndPad.NPads.Value  thermal_port=simscape.enum.thermaleffects.omit  mu_static=Vehicle.Brakes.Axle1.DiscAndPad.rMuStatic.Value  mu_coulomb=Vehicle.Brakes.Axle1.DiscAndPad.rMuKinetic.Value  temperature_TLU=[280, 300, 320] K  mu_static_TLU=[.9, .8, .7]  mu_coulomb_TLU=[.8, .7, .6]  brkwy_vel=0.1 rad/s  visc_coef=0.001 N*m/(rad/s)  thermal_mass=50 kJ/K  temperature_specify=off  temperature_priority=High  temperature=300 K  temperature_nominal_specify=off  temperature_nominal_value=1  temperature_nominal_unit=K
  Disc Brake L2 : sdl_lib/Brakes & Detents/Rotational/Disc Brake  r_mean=Vehicle.Brakes.Axle2.DiscAndPad.lMeanRadius.Value m  bore=Vehicle.Brakes.Axle2.Caliper.lCylinderDiameter.Value m  n_pads=Vehicle.Brakes.Axle2.DiscAndPad.NPads.Value  thermal_port=simscape.enum.thermaleffects.omit  mu_static=Vehicle.Brakes.Axle2.DiscAndPad.rMuStatic.Value  mu_coulomb=Vehicle.Brakes.Axle2.DiscAndPad.rMuKinetic.Value  temperature_TLU=[280, 300, 320] K  mu_static_TLU=[.9, .8, .7]  mu_coulomb_TLU=[.8, .7, .6]  brkwy_vel=0.1 rad/s  visc_coef=0.001 N*m/(rad/s)  thermal_mass=50 kJ/K  temperature_specify=off  temperature_priority=High  temperature=300 K  temperature_nominal_specify=off  temperature_nominal_value=1  temperature_nominal_unit=K
  Disc Brake R1 : sdl_lib/Brakes & Detents/Rotational/Disc Brake  r_mean=Vehicle.Brakes.Axle1.DiscAndPad.lMeanRadius.Value m  bore=Vehicle.Brakes.Axle1.Caliper.lCylinderDiameter.Value m  n_pads=Vehicle.Brakes.Axle1.DiscAndPad.NPads.Value  thermal_port=simscape.enum.thermaleffects.omit  mu_static=Vehicle.Brakes.Axle1.DiscAndPad.rMuStatic.Value  mu_coulomb=Vehicle.Brakes.Axle1.DiscAndPad.rMuKinetic.Value  temperature_TLU=[280, 300, 320] K  mu_static_TLU=[.9, .8, .7]  mu_coulomb_TLU=[.8, .7, .6]  brkwy_vel=0.1 rad/s  visc_coef=0.001 N*m/(rad/s)  thermal_mass=50 kJ/K  temperature_specify=off  temperature_priority=High  temperature=300 K  temperature_nominal_specify=off  temperature_nominal_value=1  temperature_nominal_unit=K
  Disc Brake R2 : sdl_lib/Brakes & Detents/Rotational/Disc Brake  r_mean=Vehicle.Brakes.Axle2.DiscAndPad.lMeanRadius.Value m  bore=Vehicle.Brakes.Axle2.Caliper.lCylinderDiameter.Value m  n_pads=Vehicle.Brakes.Axle2.DiscAndPad.NPads.Value  thermal_port=simscape.enum.thermaleffects.omit  mu_static=Vehicle.Brakes.Axle2.DiscAndPad.rMuStatic.Value  mu_coulomb=Vehicle.Brakes.Axle2.DiscAndPad.rMuKinetic.Value  temperature_TLU=[280, 300, 320] K  mu_static_TLU=[.9, .8, .7]  mu_coulomb_TLU=[.8, .7, .6]  brkwy_vel=0.1 rad/s  visc_coef=0.001 N*m/(rad/s)  thermal_mass=50 kJ/K  temperature_specify=off  temperature_priority=High  temperature=300 K  temperature_nominal_specify=off  temperature_nominal_value=1  temperature_nominal_unit=K
  PS Terminator{,1..3} (4 alike) : fl_lib/Physical Signals/Sinks/PS Terminator
  PS-Simulink Converter3 : nesl_utility/PS-Simulink Converter  PhysicalDomain=network_engine_domain  SubClassName=ps_output  LeftPortType=input  RightPortType=output  PseudoPeriodic=off  Frequencies=[]  VectorFormat=1-D array  Unit=m/s  AffineConversion=off
  Simulink-PS Converter{1..4} (4 alike) : nesl_utility/Simulink-PS Converter  PhysicalDomain=network_engine_domain  SubClassName=ps_input  LeftPortType=input  RightPortType=output  PseudoPeriodic=off  Frequencies=[]  NoiseDistribution=none  NoiseParameters=[]  Unit=bar  AffineConversion=off  FilteringAndDerivatives=provide  SimscapeFilterOrder=1  InputFilterTimeConstant=0.01  UdotUserProvided=0
  Tire L1 : sdl_lib/Tires & Vehicles/Tire (Magic Formula)  parameterization=1  F_z1=3000 N  F_x1=3500 N  kappa1=6  B_m=10  C_m=1.9  D_m=1  E_m=0.97  fz0=4e+3 N  p_Cx=1.685  p_Dx=[ 1.21 -0.037 ]  p_Ex=[ 0.344 0.095 -0.02 0 ]  p_Kx=[ 21.51 -0.163 0.245 ]  p_Hx=[ -0.002 0.002 ]  p_Vx=[ 0 0 ]  rolling_radius_model=sdl.enum.RollingRadiusParameterization.Constant  r_e=Vehicle.Chassis.TireA1.tire_radius.Value m  r_0=0.3 m  breff=8.39  dreff=0.26  freff=0.074  q_re0=0.99  q_v1=0.008  longvl=17 m/s  cz=5e5 N/m  model_resistance=1  resistance_model=1  coeff=0.015  p_tire=250e3 Pa  alpha=-0.003  beta=0.97  coeff_a=84e-4  coeff_b=6.2e-4 s/m  coeff_c=1.6e-4 s^2/m^2  p_tire0=240e3 Pa  fz0_resistance=4000 N  vH0=16 m/s  q_Sy=[.0082, 0, .0014, .001, 0, 0, 1.08, -.5]  v_thr=1e-3 m/s  enable_scaling_coefficients=false  lfzO=1  lcx=1  lmux=1  lex=1  lkx=1  lhx=1  lvx=1  lmy=1  model_compliance=0  stiffness=1e+6 N/m  damping=1000 N/(m/s)  model_inertia=1  inertia=Vehicle.Chassis.TireA1.Inertia.Value(1) kg*m^2  initial_velocity=Init.Axle1.nWheel.Value(1) rad/s  vxlow=0.1 m/s  v_tr_thr=0.1*(0.1) m/s  kpumin=-1e5  kpumax=1e5
  Tire L2 : sdl_lib/Tires & Vehicles/Tire (Magic Formula)  parameterization=1  F_z1=3000 N  F_x1=3500 N  kappa1=6  B_m=10  C_m=1.9  D_m=1  E_m=0.97  fz0=4e+3 N  p_Cx=1.685  p_Dx=[ 1.21 -0.037 ]  p_Ex=[ 0.344 0.095 -0.02 0 ]  p_Kx=[ 21.51 -0.163 0.245 ]  p_Hx=[ -0.002 0.002 ]  p_Vx=[ 0 0 ]  rolling_radius_model=sdl.enum.RollingRadiusParameterization.Constant  r_e=Vehicle.Chassis.TireA2.tire_radius.Value m  r_0=0.3 m  breff=8.39  dreff=0.26  freff=0.074  q_re0=0.99  q_v1=0.008  longvl=17 m/s  cz=5e5 N/m  model_resistance=1  resistance_model=1  coeff=0.015  p_tire=250e3 Pa  alpha=-0.003  beta=0.97  coeff_a=84e-4  coeff_b=6.2e-4 s/m  coeff_c=1.6e-4 s^2/m^2  p_tire0=240e3 Pa  fz0_resistance=4000 N  vH0=16 m/s  q_Sy=[.0082, 0, .0014, .001, 0, 0, 1.08, -.5]  v_thr=1e-3 m/s  enable_scaling_coefficients=false  lfzO=1  lcx=1  lmux=1  lex=1  lkx=1  lhx=1  lvx=1  lmy=1  model_compliance=0  stiffness=1e+6 N/m  damping=1000 N/(m/s)  model_inertia=1  inertia=Vehicle.Chassis.TireA2.Inertia.Value(1) kg*m^2  initial_velocity=Init.Axle2.nWheel.Value(1) rad/s  vxlow=0.1 m/s  v_tr_thr=0.1*(0.1) m/s  kpumin=-1e5  kpumax=1e5
  Tire R1 : sdl_lib/Tires & Vehicles/Tire (Magic Formula)  parameterization=1  F_z1=3000 N  F_x1=3500 N  kappa1=6  B_m=10  C_m=1.9  D_m=1  E_m=0.97  fz0=4e+3 N  p_Cx=1.685  p_Dx=[ 1.21 -0.037 ]  p_Ex=[ 0.344 0.095 -0.02 0 ]  p_Kx=[ 21.51 -0.163 0.245 ]  p_Hx=[ -0.002 0.002 ]  p_Vx=[ 0 0 ]  rolling_radius_model=sdl.enum.RollingRadiusParameterization.Constant  r_e=Vehicle.Chassis.TireA1.tire_radius.Value m  r_0=0.3 m  breff=8.39  dreff=0.26  freff=0.074  q_re0=0.99  q_v1=0.008  longvl=17 m/s  cz=5e5 N/m  model_resistance=1  resistance_model=1  coeff=0.015  p_tire=250e3 Pa  alpha=-0.003  beta=0.97  coeff_a=84e-4  coeff_b=6.2e-4 s/m  coeff_c=1.6e-4 s^2/m^2  p_tire0=240e3 Pa  fz0_resistance=4000 N  vH0=16 m/s  q_Sy=[.0082, 0, .0014, .001, 0, 0, 1.08, -.5]  v_thr=1e-3 m/s  enable_scaling_coefficients=false  lfzO=1  lcx=1  lmux=1  lex=1  lkx=1  lhx=1  lvx=1  lmy=1  model_compliance=0  stiffness=1e+6 N/m  damping=1000 N/(m/s)  model_inertia=1  inertia=Vehicle.Chassis.TireA1.Inertia.Value(1) kg*m^2  initial_velocity=Init.Axle1.nWheel.Value(1) rad/s  vxlow=0.1 m/s  v_tr_thr=0.1*(0.1) m/s  kpumin=-1e5  kpumax=1e5
  Tire R2 : sdl_lib/Tires & Vehicles/Tire (Magic Formula)  parameterization=1  F_z1=3000 N  F_x1=3500 N  kappa1=6  B_m=10  C_m=1.9  D_m=1  E_m=0.97  fz0=4e+3 N  p_Cx=1.685  p_Dx=[ 1.21 -0.037 ]  p_Ex=[ 0.344 0.095 -0.02 0 ]  p_Kx=[ 21.51 -0.163 0.245 ]  p_Hx=[ -0.002 0.002 ]  p_Vx=[ 0 0 ]  rolling_radius_model=sdl.enum.RollingRadiusParameterization.Constant  r_e=Vehicle.Chassis.TireA2.tire_radius.Value m  r_0=0.3 m  breff=8.39  dreff=0.26  freff=0.074  q_re0=0.99  q_v1=0.008  longvl=17 m/s  cz=5e5 N/m  model_resistance=1  resistance_model=1  coeff=0.015  p_tire=250e3 Pa  alpha=-0.003  beta=0.97  coeff_a=84e-4  coeff_b=6.2e-4 s/m  coeff_c=1.6e-4 s^2/m^2  p_tire0=240e3 Pa  fz0_resistance=4000 N  vH0=16 m/s  q_Sy=[.0082, 0, .0014, .001, 0, 0, 1.08, -.5]  v_thr=1e-3 m/s  enable_scaling_coefficients=false  lfzO=1  lcx=1  lmux=1  lex=1  lkx=1  lhx=1  lvx=1  lmy=1  model_compliance=0  stiffness=1e+6 N/m  damping=1000 N/(m/s)  model_inertia=1  inertia=Vehicle.Chassis.TireA2.Inertia.Value(1) kg*m^2  initial_velocity=Init.Axle2.nWheel.Value(1) rad/s  vxlow=0.1 m/s  v_tr_thr=0.1*(0.1) m/s  kpumin=-1e5  kpumax=1e5
  Transfer Fcn3 : TransferFcn  Denominator=[.001 1]
  Vehicle Body : sdl_lib/Tires & Vehicles/Vehicle Body  mass=Vehicle.Chassis.Body.m.Value kg  n_w=2  x_f=Vehicle.Chassis.Body.sAxle1.Value(1)-Vehicle.Chassis.Body.sCG.Value(1) m  x_r=-Vehicle.Chassis.Body.sAxle2.Value(1)+Vehicle.Chassis.Body.sCG.Value(1) m  y_c=Vehicle.Chassis.Body.sCG.Value(3)-Vehicle.Chassis.Body.sAxle1.Value(3) m  mass_var=simscape.enum.onoff.off  g=9.81 m/s^2  liftoff_warning=0  area=Vehicle.Chassis.Aero.ARef.Value m^2  Cd_var=false  Cd=Vehicle.Chassis.Aero.CD.Value  rho=1.18 kg/m^3  model_pitch=0  inertia=4000 kg*m^2  suspension_model=1  k_f=1e4 N/m  b_f=1e4 N/(m/s)  k_r=1e4 N/m  b_r=1e4 N/(m/s)  k_f_TLU=[-2000, -1000, 0, 1000, 2000] N  x_f_TLU=[-.4, -.2, 0, .2, .4] m  b_f_TLU=[-200, -100, 0, 100, 200] N  v_f_TLU=[-4, -2, 0, 2, 4] m/s  k_r_TLU=[-2000, -1000, 0, 1000, 2000] N  x_r_TLU=[-.4, -.2, 0, .2, .4] m  b_r_TLU=[-200, -100, 0, 100, 200] N  v_r_TLU=[-4, -2, 0, 2, 4] m/s  interp_method=simscape.enum.interpolation.linear  extrap_method=simscape.enum.extrapolation.linear  model_hardstop=0  upper_bound_f=.25 m  lower_bound_f=-.25 m  stop_k_f=1e6 N/m  stop_b_f=150 N/(m/s)  upper_bound_r=.25 m  lower_bound_r=-.25 m  stop_k_r=1e6 N/m  stop_b_r=150 N/(m/s)  initial_pitch=0 rad  initial_pitch_rate=0 rad/s  v_specify=on  v_priority=High  v=Init.Chassis.vChassis.Value(1) m/s  v_nominal_specify=off  v_nominal_value=1  v_nominal_unit=m/s
  L1 : PMIOPort  Side=Left
  R1 : PMIOPort  Port=2  Side=Right
  Out Bus Element : Outport  PortName=VehBus  Element=Body
  wires:
  PS-Simulink Converter3/1 -> Transfer Fcn3/1
  Transfer Fcn3/1 -> Bus Creator/1  "vx"
  In Bus Element1/1 -> Simulink-PS Converter1/1
  Bus Creator/1 -> Bus Creator1/1  "CG"
  Bus Creator1/1 -> Out Bus Element/1
  In Bus Element3/1 -> Simulink-PS Converter2/1
  In Bus Element2/1 -> Simulink-PS Converter3/1
  In Bus Element4/1 -> Simulink-PS Converter4/1
  connections:
  Disc Brake L1/LConn1 -- Simulink-PS Converter1/RConn1
  Tire L1/LConn2 -- L1/RConn1 -- Disc Brake L1/LConn2
  Tire L1/RConn1 -- PS Terminator/LConn1
  Vehicle Body/LConn2 -- PS-Simulink Converter3/LConn1
  Tire L1/LConn1 -- Tire R1/LConn1 -- Vehicle Body/RConn2
  Tire R2/RConn2 -- Tire L2/RConn2 -- Vehicle Body/LConn1 -- Tire R1/RConn2 -- Tire L1/RConn2
  Disc Brake R1/LConn2 -- Tire R1/LConn2 -- R1/RConn1
  Tire R1/RConn1 -- PS Terminator1/LConn1
  Tire L2/LConn2 -- Disc Brake L2/LConn2
  Tire R2/LConn1 -- Tire L2/LConn1 -- Vehicle Body/RConn1
  Tire R2/LConn2 -- Disc Brake R2/LConn2
  Tire L2/RConn1 -- PS Terminator2/LConn1
  Tire R2/RConn1 -- PS Terminator3/LConn1
  Simulink-PS Converter2/RConn1 -- Disc Brake L2/LConn1
  Simulink-PS Converter3/RConn1 -- Disc Brake R1/LConn1
  Simulink-PS Converter4/RConn1 -- Disc Brake R2/LConn1

== system ssc_car_fuel_cell_1motor/Vehicle/Powertrain ==
  VehB : Inport
  CtrlP : Inport  Port=2
  Driveline : Subsystem
      mask Display: image('ssc_vehicle_fuel_cell_1motor_driveline_IMAGE.png');
  FuelCell1Motor : Subsystem  VariantControl=FuelCell1Motor  mask(Single Motor Fuel Cell Powertrain){Power=Powertrain.Power}
      mask prompts: Power "Power (structure)"
      mask help: Models a single motor powered by fuel cell and battery.
      mask Display: image('sm_car_vehicle_power_fc1motor_IMAGE.png');
  L1 : PMIOPort  Side=Left
  R1 : PMIOPort  Port=2  Side=Right
  OutP : Outport  VectorParamsAs1DForOutWhenUnconnected=off
  wires:
  FuelCell1Motor/1(OutP) -> OutP/1
  CtrlP/1 -> FuelCell1Motor/1(CtrlBus)
  VehB/1 -> FuelCell1Motor/2(VehBus)
  connections:
  FuelCell1Motor/LConn1 -- Driveline/LConn2
  L1/RConn1 -- Driveline/LConn1
  R1/RConn1 -- Driveline/RConn1

== system ssc_car_fuel_cell_1motor/Driver/Drive Cycle/Drive Cycle Data ==
  1-D Lookup Table : Lookup_n-D  NumberOfTableDimensions=1  BreakpointsForDimension1=Drive_Cycle_Time  Table=Drive_Cycle_Speed  InterpMethod=Akima spline  InternalRulePriority=Speed  RndMeth=Simplest
  Clock : Clock
  "kmh to mps " : Gain  Gain=1/3.6
  Reference Speed : Outport  VectorParamsAs1DForOutWhenUnconnected=off
  wires:
  Clock/1 -> 1-D Lookup Table/1
  1-D Lookup Table/1 -> "kmh to mps "/1
  "kmh to mps "/1 -> Reference Speed/1  "vTarget"

== system ssc_car_fuel_cell_1motor/Driver/Vehicle Speed Controller/Configurable ==
  Ref Spd : Inport
  Veh Spd : Inport  Port=2
  Constant : Constant  Value=0
  Longitudinal Driver : autolibshared/Longitudinal Driver  extAccelOvr=off  extDecelOvr=off  extAccelHld=off  extDecelHld=off  extAccelZero=off  extDecelZero=off  cntrlType=PI  shftType=None  velUnits=km/h  gearOut=off  Kp=Driver.Long.Kp.Value/2  Ki=Driver.Long.Ki.Value/2/2  Kff=0  Kg=0  VehVelVec=[0 100]  KffVec=[.1 .1]  KpVec=[10 10]  KiVec=[5 5]  KgVec=[0 0]  m=1500  Kpt=3000  tau=.1  L=2  aR=200  bR=2.5  cR=.5  g=9.81  vnom=1  Kaw=0  tauerr=0  tauPt=2  GearInit=0  tShift=.1  pdlVec=[0.1 0.4 0.5 0.9]  upShftTbl=[-1 12.9375 26.4375 39.9375 51.18749999999999 62.4375 72.84375 83.25;-1 16.3125 29.8125 43.3125 54.5624 65.8125 76.78125 87.75;-1 19.6875 33.1875 46.68749999999999 57.9375 69.1875 80.71875 92.25;-1 33 52.5 77.25 100.5 138.75 161.875 185]  dwnShftTbl=[1 9.5625 23.0625 36.5625 47.8125 59.0625 68.90625 78.75;1 12.9375 26.4375 39.9375 51.18749999999999 62.4375 72.84375 83.25;1 16.3125 29.8125 43.3125 54.562499 65.8125 76.78125 87.75;1 19.6875 33.1875 46.68749999999999 57.9375 69.1875 80.71875 92.25]  tClutch=.5  tRev=.5  tPark=120  aMode=1  UpGearVec="[0  1  2  3  4  5  6  7]"  DownGearVec="[1  2  3  4  5  6  7  8]"
  Terminator : Terminator
  rBrakePedal : Outport  VectorParamsAs1DForOutWhenUnconnected=off
  rAccelPedal : Outport  Port=2  VectorParamsAs1DForOutWhenUnconnected=off
  wires:
  Longitudinal Driver/3 -> rBrakePedal/1  "rBrakePedal"
  Longitudinal Driver/2 -> rAccelPedal/1  "rAccelPedal"
  Constant/1 -> Longitudinal Driver/3
  Veh Spd/1 -> Longitudinal Driver/2
  Longitudinal Driver/1 -> Terminator/1
  Ref Spd/1 -> Longitudinal Driver/1

== system ssc_car_fuel_cell_1motor/Driver/Vehicle Speed Controller/Ideal ==
  Ref Spd : Inport
  Veh Spd : Inport  Port=2
  Integrator : Integrator  UpperSaturationLimit=1  LowerSaturationLimit=-1  ZeroCross=off
  Ki : Gain  Gain=Driver.Long.Ki.Value/2/2
  Kp : Gain  Gain=Driver.Long.Kp.Value/2
  Limit Acc : Saturate  UpperLimit=1  LowerLimit=0  ZeroCross=off
  Limit Brk : Saturate  UpperLimit=1  LowerLimit=0  ZeroCross=off
  Meas Lowpass Filter : TransferFcn  Denominator=[1/Driver.Filter.Measured.Value 1]
  Negative : Gain  Gain=-1
  Ref Lowpass Filter : TransferFcn  Denominator=[1/Driver.Filter.Reference.Value 1]
  Sum : Sum  Inputs=-+|
  Sum1 : Sum  Inputs=++|
  rBrakePedal : Outport  VectorParamsAs1DForOutWhenUnconnected=off
  rAccelPedal : Outport  Port=2  VectorParamsAs1DForOutWhenUnconnected=off
  wires:
  Ref Lowpass Filter/1 -> Sum/2
  Ref Spd/1 -> Ref Lowpass Filter/1
  Negative/1 -> Limit Brk/1
  Meas Lowpass Filter/1 -> Sum/1
  Limit Brk/1 -> rBrakePedal/1  "rBrakePedal"
  Veh Spd/1 -> Meas Lowpass Filter/1
  Integrator/1 -> Sum1/1
  Kp/1 -> Sum1/2
  Ki/1 -> Integrator/1
  Sum/1 -> Kp/1, Ki/1
  Sum1/1 -> Limit Acc/1, Negative/1
  Limit Acc/1 -> rAccelPedal/1  "rAccelPedal"

== system ssc_car_fuel_cell_1motor/Fuel Cell 1 Motor/FC Control/sigmoid ==
  FCpower : Inport
  Add : Sum
  Add1 : Sum  Inputs=+-
  Constant1 : Constant
  Constant2 : Constant
  Divide : Product  Inputs=*/
  Gain2 : Gain  Gain=-.001
  Math Function : Math  SignedPower=on
  optFCpower : Constant  Value=6.5e3
  multiplier : Outport
  wires:
  Constant1/1 -> Divide/1
  Gain2/1 -> Math Function/1
  FCpower/1 -> Add1/1
  Constant2/1 -> Add/1
  optFCpower/1 -> Add1/2
  Add/1 -> Divide/2
  Math Function/1 -> Add/2
  Divide/1 -> multiplier/1
  Add1/1 -> Gain2/1

== system ssc_car_fuel_cell_1motor/Fuel Cell 1 Motor/Regen Torque Limit/Check Within Limits ==
  up : Inport
  u : Inport  Port=2
  lo : Inport  Port=3
  Compare To Zero : simulink/Logic and Bit Operations/Compare To Zero  relop=>=  OutDataTypeStr=boolean
  Compare To Zero1 : simulink/Logic and Bit Operations/Compare To Zero  relop=<=  OutDataTypeStr=boolean
  Logical Operator : Logic  AllPortsSameDT=off  OutDataTypeStr=boolean
  Saturation Dynamic1 : sl_discontinuities/Saturation Dynamic  OutMin=[]  OutMax=[]  OutDataTypeStr=Inherit: Same as second input  OutDataType=fixdt(1, 16)  OutScaling=2^-10  DoSatur=off
  Subtract : Sum  Inputs=+-
  Subtract1 : Sum  Inputs=-+
  InLimit : Outport  SampleTime=0  VectorParamsAs1DForOutWhenUnconnected=off
  y : Outport  Port=2  VectorParamsAs1DForOutWhenUnconnected=off
  wires:
  Saturation Dynamic1/1 -> y/1
  lo/1 -> Subtract1/2, Saturation Dynamic1/3
  up/1 -> Subtract/1, Saturation Dynamic1/1
  u/1 -> Subtract1/1, Subtract/2, Saturation Dynamic1/2
  Subtract/1 -> Compare To Zero/1
  Subtract1/1 -> Compare To Zero1/1
  Compare To Zero/1 -> Logical Operator/1
  Compare To Zero1/1 -> Logical Operator/2
  Logical Operator/1 -> InLimit/1
